simulink model "ovenModel"  (R2020a)
settings: Solver=ode4  StartTime=0.0  StopTime=10000  FixedStep=0.01  RelTol=1e-3  EnableMultiTasking=on
undefined symbols (not defined in the file): Cg, Cs, k, kc, kg, kr, sCon, Ta, u0
settings Model: Creator=tanzc  LastModifiedBy=tanzc
settings DataIOCC: LimitDataPoints=on  SaveFormat=StructureWithTime  ReturnWorkspaceOutputs=off
settings ModelReferenceCC: EnableParallelModelReferenceBuilds=on  PropagateSignalLabelsOutOfModel=off

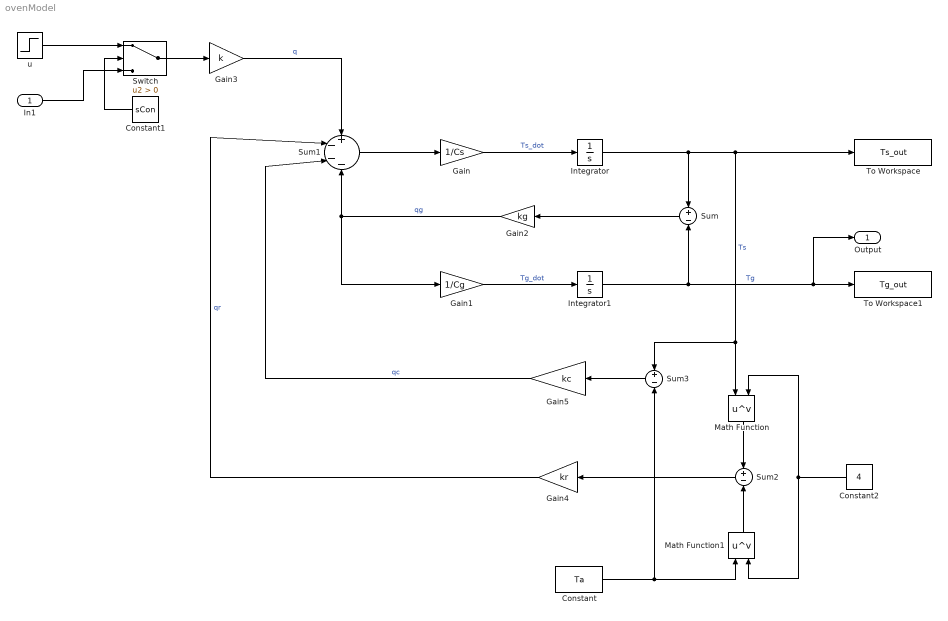
== system ovenModel ==
  In1 : Inport
  Constant : Constant  Value=Ta
  Constant1 : Constant  Value=sCon
  Constant2 : Constant  Value=4
  Gain : Gain  Gain=1/Cs
  Gain1 : Gain  Gain=1/Cg
  Gain2 : Gain  Gain=kg
  Gain3 : Gain  Gain=k
  Gain4 : Gain  Gain=kr
  Gain5 : Gain  Gain=kc
  Integrator : Integrator  Priority=1  InitialCondition=473.15
  Integrator1 : Integrator  Priority=2  InitialCondition=298.15
  Math Function : Math  Operator=pow  SignedPower=on  SaturateOnIntegerOverflow=on
  Math Function1 : Math  Operator=pow  SignedPower=on  SaturateOnIntegerOverflow=on
  Sum : Sum  Inputs=+|-
  Sum1 : Sum  Inputs=+---
  Sum2 : Sum  Inputs=+|-
  Sum3 : Sum  Inputs=+|-
  Switch : Switch  Criteria=u2 > Threshold
  To Workspace : ToWorkspace  VariableName=Ts_out  SaveFormat=Structure With Time  SampleTime=-1
  To Workspace1 : ToWorkspace  VariableName=Tg_out  SaveFormat=Structure With Time  SampleTime=-1
  u : Step  Before=u0  After=u0  SampleTime=0
  Output : Outport
  wires:
  Gain/1 -> Integrator/1  "Ts_dot"
  Integrator/1 -> Sum/1, To Workspace/1, Math Function/1, Sum3/1  "Ts"
  Integrator1/1 -> Output/1, To Workspace1/1, Sum/2  "Tg"
  Gain1/1 -> Integrator1/1  "Tg_dot"
  Sum/1 -> Gain2/1
  Gain2/1 -> Gain1/1, Sum1/4  "qg"
  Gain3/1 -> Sum1/1  "q"
  Sum1/1 -> Gain/1
  Gain5/1 -> Sum1/3  "qc"
  Constant2/1 -> Math Function1/2, Math Function/2
  Constant/1 -> Sum3/2, Math Function1/1
  Math Function/1 -> Sum2/1
  Math Function1/1 -> Sum2/2
  Sum2/1 -> Gain4/1
  Gain4/1 -> Sum1/2  "qr"
  Sum3/1 -> Gain5/1
  u/1 -> Switch/1
  In1/1 -> Switch/3
  Constant1/1 -> Switch/2
  Switch/1 -> Gain3/1
